simulink model "untitled"  (R2021b)
settings: Solver=VariableStepAuto  StartTime=0.0  StopTime=10.0  RelTol=1e-3
settings Model: Creator=Oskar  LastModifiedBy=Oskar

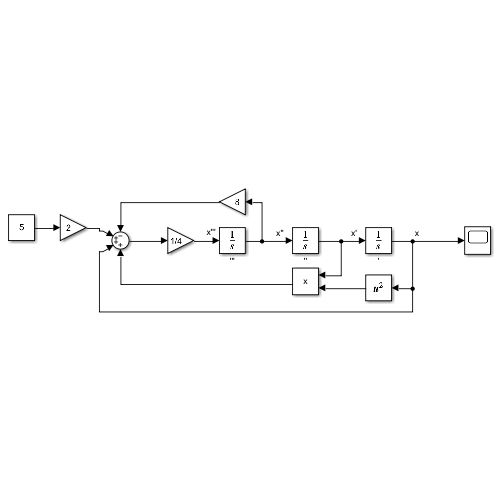
[thumbnail: Simulink's stored preview of the top-level diagram]
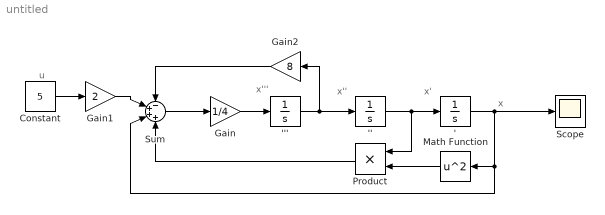
== system untitled ==
  note: x
  note: x'
  note: x''
  note: x'''
  note: u
  ' : Integrator  InitialCondition=3
  '' : Integrator  InitialCondition=1
  ''' : Integrator
  Constant : Constant  Value=5
  Gain : Gain  Gain=1/4
  Gain1 : Gain  Gain=2
  Gain2 : Gain  Gain=8
  Math Function : Math  Operator=square  SaturateOnIntegerOverflow=on
  Product : Product
  Scope : Scope
  Sum : Sum  Inputs=-+++
  wires:
  Gain/1 -> '''/1
  Sum/1 -> Gain/1
  Gain1/1 -> Sum/2
  Constant/1 -> Gain1/1
  '''/1 -> ''/1, Gain2/1
  ''/1 -> Product/1, '/1
  '/1 -> Math Function/1, Sum/3, Scope/1
  Gain2/1 -> Sum/1
  Math Function/1 -> Product/2
  Product/1 -> Sum/4
